simulink model "subsystem_118_bus"  (R2025b)
settings: Solver=ode45  StartTime=0.0  StopTime=Tstop  FixedStep=Ts  RelTol=1e-12  AbsTol=1e-12
values from neighbouring files (symbols this model uses):
  Imax = 15    [config_file.m]
  nominalInter =     [nominalInter.mat]
  nominalU =     [nominalU.mat]
  nominalY =     [nominalY.mat]
  sub = struct    [main_sub_118_bus.m]
  sys_j = sys_j(1:end-1)    [IBR_modelGenerator.m]
  sys_j_AA = sys_j    [modularMOR_main.m]
  sys_j_BT = sys_j    [modularMOR_main.m]
  Tstep_gfl = 0.1    [main_sub_118_bus.m]
  Tstep_gfm = 0.1    [main_sub_118_bus.m]
  w = 2*pi*50    (= 314.159265359)    [config_file.m]    (also in mirrorMimoWeightedFrequencyData.m = w(:); modularMOR_main.m = w(:).'; plotTest.m = w(:).')
undefined symbols (not defined in the file or in its folder): con_sub, linSys1, linSys2, linSys3
libraries: simulink x10
(part 2 of 6)

== system subsystem_118_bus/Linear 118 Bus ROM/Subsystem3/con13 ==
  In1 : Inport
  In2 : Inport  Port=2
  Constant : Constant  Value=con_subsystem.T
  Constant1 : Constant  Value=con_subsystem.T
  Mux : Mux  Inputs=2
  Selector : Selector  NumberOfDimensions=2  InputPortWidth=3  IndexOptions=Index vector (dialog),Select all  Indices=con_subsystem.reorder_v',1  OutputSizes=1,1
  Selector1 : Selector  InputPortWidth=con_subsystem.nbus  IndexOptions=Index vector (dialog)  Indices=con_subsystem.I_select{1}'  OutputSizes=1
  Selector2 : Selector  InputPortWidth=con_subsystem.nbus  IndexOptions=Index vector (dialog)  Indices=con_subsystem.I_select{3}'  OutputSizes=1
  T'x(v_bus_DQ) : Product  Multiplication=Matrix(*)
  Transpose : Math  Operator=transpose
  Tx(i_line_DQ) : Product  Multiplication=Matrix(*)
  branch RL dynamics : Subsystem
      mask Display: image('$imagefile'); % Use "Edit Image" on toolstrip to change.
  Out1 : Outport
  Out2 : Outport  Port=2
  wires:
  In2/1 -> Mux/2
  Selector2/1 -> Out2/1
  In1/1 -> Mux/1
  Selector1/1 -> Out1/1
  T'x(v_bus_DQ)/1 -> branch RL dynamics/1(v_diff_DQ)
  branch RL dynamics/1(i_line_DQ) -> Tx(i_line_DQ)/2
  Constant1/1 -> Tx(i_line_DQ)/1
  Transpose/1 -> T'x(v_bus_DQ)/1
  Constant/1 -> Transpose/1
  Tx(i_line_DQ)/1 -> Selector1/1, Selector2/1
  Selector/1 -> T'x(v_bus_DQ)/2
  Mux/1 -> Selector/1

== system subsystem_118_bus/Subsystem1/area1/branch RL dynamics ==
  v_diff_DQ : Inport
  " " : Integrator  InitialCondition=Subsystem.line.i_D  ContinuousStateAttributes='lineiD'
  -R/L : Gain  Gain=-Subsystem.line.r./Subsystem.line.l
  "-R/L " : Gain  Gain=-Subsystem.line.r./Subsystem.line.l
  1/L : Gain  Gain=1./Subsystem.line.l
  "1/L " : Gain  Gain=1./Subsystem.line.l
  Complex to Real-Imag : ComplexToRealImag
  Constant : Constant  Value=w
  Integrator1 : Integrator  InitialCondition=Subsystem.line.i_Q  ContinuousStateAttributes='lineiQ'
  Product : Product
  Product1 : Product
  Real-Imag to Complex : RealImagToComplex
  Sum2 : Sum  Inputs=+++
  Sum3 : Sum  Inputs=-++
  i_line_DQ : Outport
  wires:
  Sum2/1 -> " "/1
  Sum3/1 -> Integrator1/1
  Product/1 -> Sum2/3
  "1/L "/1 -> Sum3/2
  Product1/1 -> Sum3/1
  1/L/1 -> Sum2/2
  -R/L/1 -> Sum2/1
  "-R/L "/1 -> Sum3/3
  Integrator1/1 -> Real-Imag to Complex/2, Product/2, "-R/L "/1
  " "/1 -> Real-Imag to Complex/1, Product1/1, -R/L/1
  v_diff_DQ/1 -> Complex to Real-Imag/1
  Complex to Real-Imag/1 -> 1/L/1
  Complex to Real-Imag/2 -> "1/L "/1
  Real-Imag to Complex/1 -> i_line_DQ/1
  Constant/1 -> Product1/2, Product/1

== system subsystem_118_bus/Subsystem1/area1/bus reordering ==
  In1 : Inport
  In2 : Inport  Port=2
  Mux : Mux  Inputs=2
  Selector : Selector  NumberOfDimensions=2  InputPortWidth=3  IndexOptions=Index vector (dialog),Select all  Indices=Subsystem.reordering',1  OutputSizes=1,1
  v_bus_DQ : Outport
  wires:
  In2/1 -> Mux/2
  In1/1 -> Mux/1
  Mux/1 -> Selector/1
  Selector/1 -> v_bus_DQ/1

== system subsystem_118_bus/Subsystem1/area1/ibr ==
  I_bus_DQ : Inport
  Inport : Inport  Port=2
  Inport1 : Inport  Port=3
  Inport2 : Inport  Port=4
  Inport3 : Inport  Port=5
  Complex to Real-Imag : ComplexToRealImag
  Mux : Mux  Inputs=2
  Mux1 : Mux  Inputs=2
  Real-Imag to Complex : RealImagToComplex
  gfl : Subsystem
      mask Display: image('$imagefile'); % Use "Edit Image" on toolstrip to change.
  gfm : Subsystem  Commented=on
      mask Display: image('$imagefile'); % Use "Edit Image" on toolstrip to change.
  ibr device selector : Selector  InputPortWidth=Subsystem.total_devices.ibr  IndexOptions=Index vector (dialog)  Indices=Subsystem.device_selector.ibr  OutputSizes=1
  "ibr device selector " : Selector  InputPortWidth=Subsystem.total_devices.ibr  IndexOptions=Index vector (dialog)  Indices=Subsystem.device_selector.ibr  OutputSizes=1
  v_ibr_DQ : Outport
  Pm : Outport  Port=2
  Vm : Outport  Port=3
  Pm1 : Outport  Port=4
  Vm1 : Outport  Port=5
  wires:
  [v_gfl_pv_D] -> Mux/1
  [v_gfl_pv_Q] -> Mux1/1
  gfl/2(v_gfl_pv_Q) -> [v_gfl_pv_Q]
  gfm/1(v_gfm_pv_D) -> [v_gfm_D]
  gfm/2(v_gfm_pv_Q) -> [v_gfm_Q]
  Mux/1 -> ibr device selector/1
  Mux1/1 -> "ibr device selector "/1
  ibr device selector/1 -> Real-Imag to Complex/1
  "ibr device selector "/1 -> Real-Imag to Complex/2
  I_bus_DQ/1 -> Complex to Real-Imag/1
  Real-Imag to Complex/1 -> v_ibr_DQ/1
  Complex to Real-Imag/2 -> gfm/2(i_bus_Q), gfl/2(i_bus_Q)
  Complex to Real-Imag/1 -> gfm/1(i_bus_D), gfl/1(i_bus_D)
  gfl/1(vgfl_pv_D) -> [v_gfl_pv_D]
  [v_gfm_D] -> Mux/2
  [v_gfm_Q] -> Mux1/2
  Inport/1 -> gfl/3(Inport)
  Inport1/1 -> gfl/4(Inport1)
  gfl/4(Outport1) -> Vm/1
  gfl/3(Outport) -> Pm/1
  gfm/3(Outport) -> Pm1/1
  gfm/4(Outport1) -> Vm1/1
  Inport3/1 -> gfm/4(Inport1)
  Inport2/1 -> gfm/3(Inport)

== system subsystem_118_bus/Subsystem1/area1/non_ibr ==
  i_bus_DQ : Inport
  Complex to Real-Imag : ComplexToRealImag
  Mux : Mux  Inputs=3
  Mux1 : Mux  Inputs=3
  Real-Imag to Complex : RealImagToComplex
  floating buses : Subsystem
      mask Display: image('$imagefile'); % Use "Edit Image" on toolstrip to change.
  infinite bus : Subsystem  Commented=on
      mask Display: image('$imagefile'); % Use "Edit Image" on toolstrip to change.
  load buses : Subsystem
      mask Display: image('$imagefile'); % Use "Edit Image" on toolstrip to change.
  nonibr device selector : Selector  InputPortWidth=Subsystem.total_devices.nonibr  IndexOptions=Index vector (dialog)  Indices=Subsystem.device_selector.nonibr  OutputSizes=1
  "nonibr device selector " : Selector  InputPortWidth=Subsystem.total_devices.nonibr  IndexOptions=Index vector (dialog)  Indices=Subsystem.device_selector.nonibr  OutputSizes=1
  v_nonibr_DQ : Outport
  wires:
  infinite bus/1(Out1) -> [v_inf_D]
  infinite bus/2(Out2) -> [v_inf_Q]
  floating buses/1(v_float_D) -> [v_float_D]
  floating buses/2(v_float_Q) -> [v_float_Q]
  [v_inf_D] -> Mux/1
  Mux1/1 -> "nonibr device selector "/1
  [v_float_Q] -> Mux1/2
  [v_inf_Q] -> Mux1/1
  [v_float_D] -> Mux/2
  Mux/1 -> nonibr device selector/1
  nonibr device selector/1 -> Real-Imag to Complex/1
  "nonibr device selector "/1 -> Real-Imag to Complex/2
  Real-Imag to Complex/1 -> v_nonibr_DQ/1
  i_bus_DQ/1 -> Complex to Real-Imag/1
  Complex to Real-Imag/1 -> load buses/1(In1), floating buses/1(In1)
  Complex to Real-Imag/2 -> load buses/2(In2), floating buses/2(In2)
  load buses/2(Out2) -> [v_load_Q]
  load buses/1(Out1) -> [v_load_D]
  [v_load_D] -> Mux/3
  [v_load_Q] -> Mux1/3

== system subsystem_118_bus/Subsystem1/con12/branch RL dynamics ==
  v_diff_DQ : Inport
  " " : Integrator  InitialCondition=con_subsystem.line.i_D  ContinuousStateAttributes='lineiD'
  -R/L : Gain  Gain=-con_subsystem.line.r./con_subsystem.line.l
  "-R/L " : Gain  Gain=-con_subsystem.line.r./con_subsystem.line.l
  1/L : Gain  Gain=1./con_subsystem.line.l
  "1/L " : Gain  Gain=1./con_subsystem.line.l
  Complex to Real-Imag : ComplexToRealImag
  Constant : Constant  Value=w
  Integrator1 : Integrator  InitialCondition=con_subsystem.line.i_Q  ContinuousStateAttributes='lineiQ'
  Product : Product
  Product1 : Product
  Real-Imag to Complex : RealImagToComplex
  Sum2 : Sum  Inputs=+++
  Sum3 : Sum  Inputs=-++
  i_line_DQ : Outport
  wires:
  Sum2/1 -> " "/1
  Sum3/1 -> Integrator1/1
  Product/1 -> Sum2/3
  "1/L "/1 -> Sum3/2
  Product1/1 -> Sum3/1
  1/L/1 -> Sum2/2
  -R/L/1 -> Sum2/1
  "-R/L "/1 -> Sum3/3
  Integrator1/1 -> Real-Imag to Complex/2, Product/2, "-R/L "/1
  " "/1 -> Real-Imag to Complex/1, Product1/1, -R/L/1
  v_diff_DQ/1 -> Complex to Real-Imag/1
  Complex to Real-Imag/1 -> 1/L/1
  Complex to Real-Imag/2 -> "1/L "/1
  Real-Imag to Complex/1 -> i_line_DQ/1
  Constant/1 -> Product1/2, Product/1

== system subsystem_118_bus/Subsystem2/area2/branch RL dynamics ==
  v_diff_DQ : Inport
  " " : Integrator  InitialCondition=Subsystem.line.i_D  ContinuousStateAttributes='lineiD'
  -R/L : Gain  Gain=-Subsystem.line.r./Subsystem.line.l
  "-R/L " : Gain  Gain=-Subsystem.line.r./Subsystem.line.l
  1/L : Gain  Gain=1./Subsystem.line.l
  "1/L " : Gain  Gain=1./Subsystem.line.l
  Complex to Real-Imag : ComplexToRealImag
  Constant : Constant  Value=w
  Integrator1 : Integrator  InitialCondition=Subsystem.line.i_Q  ContinuousStateAttributes='lineiQ'
  Product : Product
  Product1 : Product
  Real-Imag to Complex : RealImagToComplex
  Sum2 : Sum  Inputs=+++
  Sum3 : Sum  Inputs=-++
  i_line_DQ : Outport
  wires:
  Constant/1 -> Product/1, Product1/2
  Real-Imag to Complex/1 -> i_line_DQ/1
  Complex to Real-Imag/2 -> "1/L "/1
  Complex to Real-Imag/1 -> 1/L/1
  v_diff_DQ/1 -> Complex to Real-Imag/1
  " "/1 -> -R/L/1, Product1/1, Real-Imag to Complex/1
  Integrator1/1 -> "-R/L "/1, Product/2, Real-Imag to Complex/2
  "-R/L "/1 -> Sum3/3
  -R/L/1 -> Sum2/1
  1/L/1 -> Sum2/2
  Product1/1 -> Sum3/1
  "1/L "/1 -> Sum3/2
  Product/1 -> Sum2/3
  Sum3/1 -> Integrator1/1
  Sum2/1 -> " "/1

== system subsystem_118_bus/Subsystem2/area2/bus reordering ==
  In1 : Inport
  In2 : Inport  Port=2
  Mux : Mux  Inputs=2
  Selector : Selector  NumberOfDimensions=2  InputPortWidth=3  IndexOptions=Index vector (dialog),Select all  Indices=Subsystem.reordering',1  OutputSizes=1,1
  v_bus_DQ : Outport
  wires:
  Selector/1 -> v_bus_DQ/1
  Mux/1 -> Selector/1
  In1/1 -> Mux/1
  In2/1 -> Mux/2

== system subsystem_118_bus/Subsystem2/area2/ibr ==
  I_bus_DQ : Inport
  Inport : Inport  Port=2
  Inport1 : Inport  Port=3
  Inport2 : Inport  Port=4
  Inport3 : Inport  Port=5
  Complex to Real-Imag : ComplexToRealImag
  Mux : Mux  Inputs=2
  Mux1 : Mux  Inputs=2
  Real-Imag to Complex : RealImagToComplex
  gfl : Subsystem
      mask Display: image('$imagefile'); % Use "Edit Image" on toolstrip to change.
  gfm : Subsystem
      mask Display: image('$imagefile'); % Use "Edit Image" on toolstrip to change.
  ibr device selector : Selector  InputPortWidth=Subsystem.total_devices.ibr  IndexOptions=Index vector (dialog)  Indices=Subsystem.device_selector.ibr  OutputSizes=1
  "ibr device selector " : Selector  InputPortWidth=Subsystem.total_devices.ibr  IndexOptions=Index vector (dialog)  Indices=Subsystem.device_selector.ibr  OutputSizes=1
  v_ibr_DQ : Outport
  Pm : Outport  Port=2
  Vm : Outport  Port=3
  Pm1 : Outport  Port=4
  Vm1 : Outport  Port=5
  wires:
  [v_gfl_pv_D] -> Mux/1
  [v_gfl_pv_Q] -> Mux1/1
  gfl/2(v_gfl_pv_Q) -> [v_gfl_pv_Q]
  gfm/1(v_gfm_pv_D) -> [v_gfm_D]
  gfm/2(v_gfm_pv_Q) -> [v_gfm_Q]
  Mux/1 -> ibr device selector/1
  Mux1/1 -> "ibr device selector "/1
  ibr device selector/1 -> Real-Imag to Complex/1
  "ibr device selector "/1 -> Real-Imag to Complex/2
  I_bus_DQ/1 -> Complex to Real-Imag/1
  Real-Imag to Complex/1 -> v_ibr_DQ/1
  Complex to Real-Imag/2 -> gfm/2(i_bus_Q), gfl/2(i_bus_Q)
  Complex to Real-Imag/1 -> gfm/1(i_bus_D), gfl/1(i_bus_D)
  gfl/1(vgfl_pv_D) -> [v_gfl_pv_D]
  [v_gfm_D] -> Mux/2
  [v_gfm_Q] -> Mux1/2
  Inport/1 -> gfl/3(Inport)
  Inport1/1 -> gfl/4(Inport1)
  gfl/4(Outport1) -> Vm/1
  gfl/3(Outport) -> Pm/1
  gfm/3(Outport) -> Pm1/1
  gfm/4(Outport1) -> Vm1/1
  Inport3/1 -> gfm/4(Inport1)
  Inport2/1 -> gfm/3(Inport)

== system subsystem_118_bus/Subsystem2/area2/non_ibr ==
  i_bus_DQ : Inport
  Complex to Real-Imag : ComplexToRealImag
  Mux : Mux  Inputs=3
  Mux1 : Mux  Inputs=3
  Real-Imag to Complex : RealImagToComplex
  floating buses : Subsystem
      mask Display: image('$imagefile'); % Use "Edit Image" on toolstrip to change.
  infinite bus : Subsystem  Commented=on
      mask Display: image('$imagefile'); % Use "Edit Image" on toolstrip to change.
  load buses : Subsystem
      mask Display: image('$imagefile'); % Use "Edit Image" on toolstrip to change.
  nonibr device selector : Selector  InputPortWidth=Subsystem.total_devices.nonibr  IndexOptions=Index vector (dialog)  Indices=Subsystem.device_selector.nonibr  OutputSizes=1
  "nonibr device selector " : Selector  InputPortWidth=Subsystem.total_devices.nonibr  IndexOptions=Index vector (dialog)  Indices=Subsystem.device_selector.nonibr  OutputSizes=1
  v_nonibr_DQ : Outport
  wires:
  [v_load_Q] -> Mux1/3
  [v_load_D] -> Mux/3
  load buses/1(Out1) -> [v_load_D]
  load buses/2(Out2) -> [v_load_Q]
  Complex to Real-Imag/2 -> floating buses/2(In2), load buses/2(In2)
  Complex to Real-Imag/1 -> floating buses/1(In1), load buses/1(In1)
  i_bus_DQ/1 -> Complex to Real-Imag/1
  Real-Imag to Complex/1 -> v_nonibr_DQ/1
  "nonibr device selector "/1 -> Real-Imag to Complex/2
  nonibr device selector/1 -> Real-Imag to Complex/1
  Mux/1 -> nonibr device selector/1
  [v_float_D] -> Mux/2
  [v_inf_Q] -> Mux1/1
  [v_float_Q] -> Mux1/2
  Mux1/1 -> "nonibr device selector "/1
  [v_inf_D] -> Mux/1
  floating buses/2(v_float_Q) -> [v_float_Q]
  floating buses/1(v_float_D) -> [v_float_D]
  infinite bus/2(Out2) -> [v_inf_Q]
  infinite bus/1(Out1) -> [v_inf_D]

== system subsystem_118_bus/Subsystem2/con23/branch RL dynamics ==
  v_diff_DQ : Inport
  " " : Integrator  InitialCondition=con_subsystem.line.i_D  ContinuousStateAttributes='lineiD'
  -R/L : Gain  Gain=-con_subsystem.line.r./con_subsystem.line.l
  "-R/L " : Gain  Gain=-con_subsystem.line.r./con_subsystem.line.l
  1/L : Gain  Gain=1./con_subsystem.line.l
  "1/L " : Gain  Gain=1./con_subsystem.line.l
  Complex to Real-Imag : ComplexToRealImag
  Constant : Constant  Value=w
  Integrator1 : Integrator  InitialCondition=con_subsystem.line.i_Q  ContinuousStateAttributes='lineiQ'
  Product : Product
  Product1 : Product
  Real-Imag to Complex : RealImagToComplex
  Sum2 : Sum  Inputs=+++
  Sum3 : Sum  Inputs=-++
  i_line_DQ : Outport
  wires:
  Sum2/1 -> " "/1
  Sum3/1 -> Integrator1/1
  Product/1 -> Sum2/3
  "1/L "/1 -> Sum3/2
  Product1/1 -> Sum3/1
  1/L/1 -> Sum2/2
  -R/L/1 -> Sum2/1
  "-R/L "/1 -> Sum3/3
  Integrator1/1 -> Real-Imag to Complex/2, Product/2, "-R/L "/1
  " "/1 -> Real-Imag to Complex/1, Product1/1, -R/L/1
  v_diff_DQ/1 -> Complex to Real-Imag/1
  Complex to Real-Imag/1 -> 1/L/1
  Complex to Real-Imag/2 -> "1/L "/1
  Real-Imag to Complex/1 -> i_line_DQ/1
  Constant/1 -> Product1/2, Product/1

== system subsystem_118_bus/Subsystem3/area3/branch RL dynamics ==
  v_diff_DQ : Inport
  " " : Integrator  InitialCondition=Subsystem.line.i_D  ContinuousStateAttributes='lineiD'
  -R/L : Gain  Gain=-Subsystem.line.r./Subsystem.line.l
  "-R/L " : Gain  Gain=-Subsystem.line.r./Subsystem.line.l
  1/L : Gain  Gain=1./Subsystem.line.l
  "1/L " : Gain  Gain=1./Subsystem.line.l
  Complex to Real-Imag : ComplexToRealImag
  Constant : Constant  Value=w
  Integrator1 : Integrator  InitialCondition=Subsystem.line.i_Q  ContinuousStateAttributes='lineiQ'
  Product : Product
  Product1 : Product
  Real-Imag to Complex : RealImagToComplex
  Sum2 : Sum  Inputs=+++
  Sum3 : Sum  Inputs=-++
  i_line_DQ : Outport
  wires:
  Sum2/1 -> " "/1
  Sum3/1 -> Integrator1/1
  Product/1 -> Sum2/3
  "1/L "/1 -> Sum3/2
  Product1/1 -> Sum3/1
  1/L/1 -> Sum2/2
  -R/L/1 -> Sum2/1
  "-R/L "/1 -> Sum3/3
  Integrator1/1 -> Real-Imag to Complex/2, Product/2, "-R/L "/1
  " "/1 -> Real-Imag to Complex/1, Product1/1, -R/L/1
  v_diff_DQ/1 -> Complex to Real-Imag/1
  Complex to Real-Imag/1 -> 1/L/1
  Complex to Real-Imag/2 -> "1/L "/1
  Real-Imag to Complex/1 -> i_line_DQ/1
  Constant/1 -> Product1/2, Product/1

== system subsystem_118_bus/Subsystem3/area3/bus reordering ==
  In1 : Inport
  In2 : Inport  Port=2
  Mux : Mux  Inputs=2
  Selector : Selector  NumberOfDimensions=2  InputPortWidth=3  IndexOptions=Index vector (dialog),Select all  Indices=Subsystem.reordering',1  OutputSizes=1,1
  v_bus_DQ : Outport
  wires:
  In2/1 -> Mux/2
  In1/1 -> Mux/1
  Mux/1 -> Selector/1
  Selector/1 -> v_bus_DQ/1

== system subsystem_118_bus/Subsystem3/area3/ibr ==
  I_bus_DQ : Inport
  Inport : Inport  Port=2
  Inport1 : Inport  Port=3
  Inport2 : Inport  Port=4
  Inport3 : Inport  Port=5
  Complex to Real-Imag : ComplexToRealImag
  Mux : Mux  Inputs=2
  Mux1 : Mux  Inputs=2
  Real-Imag to Complex : RealImagToComplex
  gfl : Subsystem
      mask Display: image('$imagefile'); % Use "Edit Image" on toolstrip to change.
  gfm : Subsystem  Commented=on
      mask Display: image('$imagefile'); % Use "Edit Image" on toolstrip to change.
  ibr device selector : Selector  InputPortWidth=Subsystem.total_devices.ibr  IndexOptions=Index vector (dialog)  Indices=Subsystem.device_selector.ibr  OutputSizes=1
  "ibr device selector " : Selector  InputPortWidth=Subsystem.total_devices.ibr  IndexOptions=Index vector (dialog)  Indices=Subsystem.device_selector.ibr  OutputSizes=1
  v_ibr_DQ : Outport
  Pm : Outport  Port=2
  Vm : Outport  Port=3
  Pm1 : Outport  Port=4
  Vm1 : Outport  Port=5
  wires:
  [v_gfl_pv_D] -> Mux/1
  [v_gfl_pv_Q] -> Mux1/1
  gfl/2(v_gfl_pv_Q) -> [v_gfl_pv_Q]
  gfm/1(v_gfm_pv_D) -> [v_gfm_D]
  gfm/2(v_gfm_pv_Q) -> [v_gfm_Q]
  Mux/1 -> ibr device selector/1
  Mux1/1 -> "ibr device selector "/1
  ibr device selector/1 -> Real-Imag to Complex/1
  "ibr device selector "/1 -> Real-Imag to Complex/2
  I_bus_DQ/1 -> Complex to Real-Imag/1
  Real-Imag to Complex/1 -> v_ibr_DQ/1
  Complex to Real-Imag/2 -> gfm/2(i_bus_Q), gfl/2(i_bus_Q)
  Complex to Real-Imag/1 -> gfm/1(i_bus_D), gfl/1(i_bus_D)
  gfl/1(vgfl_pv_D) -> [v_gfl_pv_D]
  [v_gfm_D] -> Mux/2
  [v_gfm_Q] -> Mux1/2
  Inport/1 -> gfl/3(Inport)
  Inport1/1 -> gfl/4(Inport1)
  gfl/4(Outport1) -> Vm/1
  gfl/3(Outport) -> Pm/1
  gfm/3(Outport) -> Pm1/1
  gfm/4(Outport1) -> Vm1/1
  Inport3/1 -> gfm/4(Inport1)
  Inport2/1 -> gfm/3(Inport)

== system subsystem_118_bus/Subsystem3/area3/non_ibr ==
  i_bus_DQ : Inport
  Complex to Real-Imag : ComplexToRealImag
  Mux : Mux  Inputs=3
  Mux1 : Mux  Inputs=3
  Real-Imag to Complex : RealImagToComplex
  floating buses : Subsystem  Commented=on
      mask Display: image('$imagefile'); % Use "Edit Image" on toolstrip to change.
  infinite bus : Subsystem  Commented=on
      mask Display: image('$imagefile'); % Use "Edit Image" on toolstrip to change.
  load buses : Subsystem
      mask Display: image('$imagefile'); % Use "Edit Image" on toolstrip to change.
  nonibr device selector : Selector  InputPortWidth=Subsystem.total_devices.nonibr  IndexOptions=Index vector (dialog)  Indices=Subsystem.device_selector.nonibr  OutputSizes=1
  "nonibr device selector " : Selector  InputPortWidth=Subsystem.total_devices.nonibr  IndexOptions=Index vector (dialog)  Indices=Subsystem.device_selector.nonibr  OutputSizes=1
  v_nonibr_DQ : Outport
  wires:
  infinite bus/1(Out1) -> [v_inf_D]
  infinite bus/2(Out2) -> [v_inf_Q]
  floating buses/1(v_float_D) -> [v_float_D]
  floating buses/2(v_float_Q) -> [v_float_Q]
  [v_inf_D] -> Mux/1
  Mux1/1 -> "nonibr device selector "/1
  [v_float_Q] -> Mux1/2
  [v_inf_Q] -> Mux1/1
  [v_float_D] -> Mux/2
  Mux/1 -> nonibr device selector/1
  nonibr device selector/1 -> Real-Imag to Complex/1
  "nonibr device selector "/1 -> Real-Imag to Complex/2
  Real-Imag to Complex/1 -> v_nonibr_DQ/1
  i_bus_DQ/1 -> Complex to Real-Imag/1
  Complex to Real-Imag/1 -> load buses/1(In1), floating buses/1(In1)
  Complex to Real-Imag/2 -> load buses/2(In2), floating buses/2(In2)
  load buses/2(Out2) -> [v_load_Q]
  load buses/1(Out1) -> [v_load_D]
  [v_load_D] -> Mux/3
  [v_load_Q] -> Mux1/3

== system subsystem_118_bus/Subsystem3/con13/branch RL dynamics ==
  v_diff_DQ : Inport
  " " : Integrator  InitialCondition=con_subsystem.line.i_D  ContinuousStateAttributes='lineiD'
  -R/L : Gain  Gain=-con_subsystem.line.r./con_subsystem.line.l
  "-R/L " : Gain  Gain=-con_subsystem.line.r./con_subsystem.line.l
  1/L : Gain  Gain=1./con_subsystem.line.l
  "1/L " : Gain  Gain=1./con_subsystem.line.l
  Complex to Real-Imag : ComplexToRealImag
  Constant : Constant  Value=w
  Integrator1 : Integrator  InitialCondition=con_subsystem.line.i_Q  ContinuousStateAttributes='lineiQ'
  Product : Product
  Product1 : Product
  Real-Imag to Complex : RealImagToComplex
  Sum2 : Sum  Inputs=+++
  Sum3 : Sum  Inputs=-++
  i_line_DQ : Outport
  wires:
  Constant/1 -> Product/1, Product1/2
  Real-Imag to Complex/1 -> i_line_DQ/1
  Complex to Real-Imag/2 -> "1/L "/1
  Complex to Real-Imag/1 -> 1/L/1
  v_diff_DQ/1 -> Complex to Real-Imag/1
  " "/1 -> -R/L/1, Product1/1, Real-Imag to Complex/1
  Integrator1/1 -> "-R/L "/1, Product/2, Real-Imag to Complex/2
  "-R/L "/1 -> Sum3/3
  -R/L/1 -> Sum2/1
  1/L/1 -> Sum2/2
  Product1/1 -> Sum3/1
  "1/L "/1 -> Sum3/2
  Product/1 -> Sum2/3
  Sum3/1 -> Integrator1/1
  Sum2/1 -> " "/1

== system subsystem_118_bus/Linear 118 Bus FOM/Subsystem3/area3/branch RL dynamics ==
  v_diff_DQ : Inport
  " " : Integrator  InitialCondition=Subsystem.line.i_D  ContinuousStateAttributes='lineiD'
  -R/L : Gain  Gain=-Subsystem.line.r./Subsystem.line.l
  "-R/L " : Gain  Gain=-Subsystem.line.r./Subsystem.line.l
  1/L : Gain  Gain=1./Subsystem.line.l
  "1/L " : Gain  Gain=1./Subsystem.line.l
  Complex to Real-Imag : ComplexToRealImag
  Constant : Constant  Value=w
  Integrator1 : Integrator  InitialCondition=Subsystem.line.i_Q  ContinuousStateAttributes='lineiQ'
  Product : Product
  Product1 : Product
  Real-Imag to Complex : RealImagToComplex
  Sum2 : Sum  Inputs=+++
  Sum3 : Sum  Inputs=-++
  i_line_DQ : Outport
  wires:
  Sum2/1 -> " "/1
  Sum3/1 -> Integrator1/1
  Product/1 -> Sum2/3
  "1/L "/1 -> Sum3/2
  Product1/1 -> Sum3/1
  1/L/1 -> Sum2/2
  -R/L/1 -> Sum2/1
  "-R/L "/1 -> Sum3/3
  Integrator1/1 -> Real-Imag to Complex/2, Product/2, "-R/L "/1
  " "/1 -> Real-Imag to Complex/1, Product1/1, -R/L/1
  v_diff_DQ/1 -> Complex to Real-Imag/1
  Complex to Real-Imag/1 -> 1/L/1
  Complex to Real-Imag/2 -> "1/L "/1
  Real-Imag to Complex/1 -> i_line_DQ/1
  Constant/1 -> Product1/2, Product/1

== system subsystem_118_bus/Linear 118 Bus FOM/Subsystem3/area3/bus reordering ==
  In1 : Inport
  In2 : Inport  Port=2
  Mux : Mux  Inputs=2
  Selector : Selector  NumberOfDimensions=2  InputPortWidth=3  IndexOptions=Index vector (dialog),Select all  Indices=Subsystem.reordering',1  OutputSizes=1,1
  v_bus_DQ : Outport
  wires:
  In2/1 -> Mux/2
  In1/1 -> Mux/1
  Mux/1 -> Selector/1
  Selector/1 -> v_bus_DQ/1

== system subsystem_118_bus/Linear 118 Bus FOM/Subsystem3/area3/ibr ==
  I_bus_DQ : Inport
  Inport : Inport  Port=2
  Inport1 : Inport  Port=3
  Inport2 : Inport  Port=4
  Inport3 : Inport  Port=5
  Complex to Real-Imag : ComplexToRealImag
  Mux : Mux  Inputs=2
  Mux1 : Mux  Inputs=2
  Real-Imag to Complex : RealImagToComplex
  gfl : Subsystem
      mask Display: image('$imagefile'); % Use "Edit Image" on toolstrip to change.
  gfm : Subsystem  Commented=on
      mask Display: image('$imagefile'); % Use "Edit Image" on toolstrip to change.
  ibr device selector : Selector  InputPortWidth=Subsystem.total_devices.ibr  IndexOptions=Index vector (dialog)  Indices=Subsystem.device_selector.ibr  OutputSizes=1
  "ibr device selector " : Selector  InputPortWidth=Subsystem.total_devices.ibr  IndexOptions=Index vector (dialog)  Indices=Subsystem.device_selector.ibr  OutputSizes=1
  v_ibr_DQ : Outport
  Pm : Outport  Port=2
  Vm : Outport  Port=3
  Pm1 : Outport  Port=4
  Vm1 : Outport  Port=5
  wires:
  [v_gfl_pv_D] -> Mux/1
  [v_gfl_pv_Q] -> Mux1/1
  gfl/2(v_gfl_pv_Q) -> [v_gfl_pv_Q]
  gfm/1(v_gfm_pv_D) -> [v_gfm_D]
  gfm/2(v_gfm_pv_Q) -> [v_gfm_Q]
  Mux/1 -> ibr device selector/1
  Mux1/1 -> "ibr device selector "/1
  ibr device selector/1 -> Real-Imag to Complex/1
  "ibr device selector "/1 -> Real-Imag to Complex/2
  I_bus_DQ/1 -> Complex to Real-Imag/1
  Real-Imag to Complex/1 -> v_ibr_DQ/1
  Complex to Real-Imag/2 -> gfm/2(i_bus_Q), gfl/2(i_bus_Q)
  Complex to Real-Imag/1 -> gfm/1(i_bus_D), gfl/1(i_bus_D)
  gfl/1(vgfl_pv_D) -> [v_gfl_pv_D]
  [v_gfm_D] -> Mux/2
  [v_gfm_Q] -> Mux1/2
  Inport/1 -> gfl/3(Inport)
  Inport1/1 -> gfl/4(Inport1)
  gfl/4(Outport1) -> Vm/1
  gfl/3(Outport) -> Pm/1
  gfm/3(Outport) -> Pm1/1
  gfm/4(Outport1) -> Vm1/1
  Inport3/1 -> gfm/4(Inport1)
  Inport2/1 -> gfm/3(Inport)

== system subsystem_118_bus/Linear 118 Bus FOM/Subsystem3/area3/non_ibr ==
  i_bus_DQ : Inport
  Complex to Real-Imag : ComplexToRealImag
  Mux : Mux  Inputs=3
  Mux1 : Mux  Inputs=3
  Real-Imag to Complex : RealImagToComplex
  floating buses : Subsystem  Commented=on
      mask Display: image('$imagefile'); % Use "Edit Image" on toolstrip to change.
  infinite bus : Subsystem  Commented=on
      mask Display: image('$imagefile'); % Use "Edit Image" on toolstrip to change.
  load buses : Subsystem
      mask Display: image('$imagefile'); % Use "Edit Image" on toolstrip to change.
  nonibr device selector : Selector  InputPortWidth=Subsystem.total_devices.nonibr  IndexOptions=Index vector (dialog)  Indices=Subsystem.device_selector.nonibr  OutputSizes=1
  "nonibr device selector " : Selector  InputPortWidth=Subsystem.total_devices.nonibr  IndexOptions=Index vector (dialog)  Indices=Subsystem.device_selector.nonibr  OutputSizes=1
  v_nonibr_DQ : Outport
  wires:
  infinite bus/1(Out1) -> [v_inf_D]
  infinite bus/2(Out2) -> [v_inf_Q]
  floating buses/1(v_float_D) -> [v_float_D]
  floating buses/2(v_float_Q) -> [v_float_Q]
  [v_inf_D] -> Mux/1
  Mux1/1 -> "nonibr device selector "/1
  [v_float_Q] -> Mux1/2
  [v_inf_Q] -> Mux1/1
  [v_float_D] -> Mux/2
  Mux/1 -> nonibr device selector/1
  nonibr device selector/1 -> Real-Imag to Complex/1
  "nonibr device selector "/1 -> Real-Imag to Complex/2
  Real-Imag to Complex/1 -> v_nonibr_DQ/1
  i_bus_DQ/1 -> Complex to Real-Imag/1
  Complex to Real-Imag/1 -> load buses/1(In1), floating buses/1(In1)
  Complex to Real-Imag/2 -> load buses/2(In2), floating buses/2(In2)
  load buses/2(Out2) -> [v_load_Q]
  load buses/1(Out1) -> [v_load_D]
  [v_load_D] -> Mux/3
  [v_load_Q] -> Mux1/3

== system subsystem_118_bus/Linear 118 Bus FOM/Subsystem3/con13/branch RL dynamics ==
  v_diff_DQ : Inport
  " " : Integrator  InitialCondition=con_subsystem.line.i_D  ContinuousStateAttributes='lineiD'
  -R/L : Gain  Gain=-con_subsystem.line.r./con_subsystem.line.l
  "-R/L " : Gain  Gain=-con_subsystem.line.r./con_subsystem.line.l
  1/L : Gain  Gain=1./con_subsystem.line.l
  "1/L " : Gain  Gain=1./con_subsystem.line.l
  Complex to Real-Imag : ComplexToRealImag
  Constant : Constant  Value=w
  Integrator1 : Integrator  InitialCondition=con_subsystem.line.i_Q  ContinuousStateAttributes='lineiQ'
  Product : Product
  Product1 : Product
  Real-Imag to Complex : RealImagToComplex
  Sum2 : Sum  Inputs=+++
  Sum3 : Sum  Inputs=-++
  i_line_DQ : Outport
  wires:
  Constant/1 -> Product/1, Product1/2
  Real-Imag to Complex/1 -> i_line_DQ/1
  Complex to Real-Imag/2 -> "1/L "/1
  Complex to Real-Imag/1 -> 1/L/1
  v_diff_DQ/1 -> Complex to Real-Imag/1
  " "/1 -> -R/L/1, Product1/1, Real-Imag to Complex/1
  Integrator1/1 -> "-R/L "/1, Product/2, Real-Imag to Complex/2
  "-R/L "/1 -> Sum3/3
  -R/L/1 -> Sum2/1
  1/L/1 -> Sum2/2
  Product1/1 -> Sum3/1
  "1/L "/1 -> Sum3/2
  Product/1 -> Sum2/3
  Sum3/1 -> Integrator1/1
  Sum2/1 -> " "/1

== system subsystem_118_bus/Linear 118 Bus ROM/Subsystem3/area3/branch RL dynamics ==
  v_diff_DQ : Inport
  " " : Integrator  InitialCondition=Subsystem.line.i_D  ContinuousStateAttributes='lineiD'
  -R/L : Gain  Gain=-Subsystem.line.r./Subsystem.line.l
  "-R/L " : Gain  Gain=-Subsystem.line.r./Subsystem.line.l
  1/L : Gain  Gain=1./Subsystem.line.l
  "1/L " : Gain  Gain=1./Subsystem.line.l
  Complex to Real-Imag : ComplexToRealImag
  Constant : Constant  Value=w
  Integrator1 : Integrator  InitialCondition=Subsystem.line.i_Q  ContinuousStateAttributes='lineiQ'
  Product : Product
  Product1 : Product
  Real-Imag to Complex : RealImagToComplex
  Sum2 : Sum  Inputs=+++
  Sum3 : Sum  Inputs=-++
  i_line_DQ : Outport
  wires:
  Sum2/1 -> " "/1
  Sum3/1 -> Integrator1/1
  Product/1 -> Sum2/3
  "1/L "/1 -> Sum3/2
  Product1/1 -> Sum3/1
  1/L/1 -> Sum2/2
  -R/L/1 -> Sum2/1
  "-R/L "/1 -> Sum3/3
  Integrator1/1 -> Real-Imag to Complex/2, Product/2, "-R/L "/1
  " "/1 -> Real-Imag to Complex/1, Product1/1, -R/L/1
  v_diff_DQ/1 -> Complex to Real-Imag/1
  Complex to Real-Imag/1 -> 1/L/1
  Complex to Real-Imag/2 -> "1/L "/1
  Real-Imag to Complex/1 -> i_line_DQ/1
  Constant/1 -> Product1/2, Product/1

== system subsystem_118_bus/Linear 118 Bus ROM/Subsystem3/area3/bus reordering ==
  In1 : Inport
  In2 : Inport  Port=2
  Mux : Mux  Inputs=2
  Selector : Selector  NumberOfDimensions=2  InputPortWidth=3  IndexOptions=Index vector (dialog),Select all  Indices=Subsystem.reordering',1  OutputSizes=1,1
  v_bus_DQ : Outport
  wires:
  In2/1 -> Mux/2
  In1/1 -> Mux/1
  Mux/1 -> Selector/1
  Selector/1 -> v_bus_DQ/1

== system subsystem_118_bus/Linear 118 Bus ROM/Subsystem3/area3/ibr ==
  I_bus_DQ : Inport
  Inport : Inport  Port=2
  Inport1 : Inport  Port=3
  Inport2 : Inport  Port=4
  Inport3 : Inport  Port=5
  Complex to Real-Imag : ComplexToRealImag
  Mux : Mux  Inputs=2
  Mux1 : Mux  Inputs=2
  Real-Imag to Complex : RealImagToComplex
  gfl : Subsystem
      mask Display: image('$imagefile'); % Use "Edit Image" on toolstrip to change.
  gfm : Subsystem  Commented=on
      mask Display: image('$imagefile'); % Use "Edit Image" on toolstrip to change.
  ibr device selector : Selector  InputPortWidth=Subsystem.total_devices.ibr  IndexOptions=Index vector (dialog)  Indices=Subsystem.device_selector.ibr  OutputSizes=1
  "ibr device selector " : Selector  InputPortWidth=Subsystem.total_devices.ibr  IndexOptions=Index vector (dialog)  Indices=Subsystem.device_selector.ibr  OutputSizes=1
  v_ibr_DQ : Outport
  Pm : Outport  Port=2
  Vm : Outport  Port=3
  Pm1 : Outport  Port=4
  Vm1 : Outport  Port=5
  wires:
  [v_gfl_pv_D] -> Mux/1
  [v_gfl_pv_Q] -> Mux1/1
  gfl/2(v_gfl_pv_Q) -> [v_gfl_pv_Q]
  gfm/1(v_gfm_pv_D) -> [v_gfm_D]
  gfm/2(v_gfm_pv_Q) -> [v_gfm_Q]
  Mux/1 -> ibr device selector/1
  Mux1/1 -> "ibr device selector "/1
  ibr device selector/1 -> Real-Imag to Complex/1
  "ibr device selector "/1 -> Real-Imag to Complex/2
  I_bus_DQ/1 -> Complex to Real-Imag/1
  Real-Imag to Complex/1 -> v_ibr_DQ/1
  Complex to Real-Imag/2 -> gfm/2(i_bus_Q), gfl/2(i_bus_Q)
  Complex to Real-Imag/1 -> gfm/1(i_bus_D), gfl/1(i_bus_D)
  gfl/1(vgfl_pv_D) -> [v_gfl_pv_D]
  [v_gfm_D] -> Mux/2
  [v_gfm_Q] -> Mux1/2
  Inport/1 -> gfl/3(Inport)
  Inport1/1 -> gfl/4(Inport1)
  gfl/4(Outport1) -> Vm/1
  gfl/3(Outport) -> Pm/1
  gfm/3(Outport) -> Pm1/1
  gfm/4(Outport1) -> Vm1/1
  Inport3/1 -> gfm/4(Inport1)
  Inport2/1 -> gfm/3(Inport)

== system subsystem_118_bus/Linear 118 Bus ROM/Subsystem3/area3/non_ibr ==
  i_bus_DQ : Inport
  Complex to Real-Imag : ComplexToRealImag
  Mux : Mux  Inputs=3
  Mux1 : Mux  Inputs=3
  Real-Imag to Complex : RealImagToComplex
  floating buses : Subsystem  Commented=on
      mask Display: image('$imagefile'); % Use "Edit Image" on toolstrip to change.
  infinite bus : Subsystem  Commented=on
      mask Display: image('$imagefile'); % Use "Edit Image" on toolstrip to change.
  load buses : Subsystem
      mask Display: image('$imagefile'); % Use "Edit Image" on toolstrip to change.
  nonibr device selector : Selector  InputPortWidth=Subsystem.total_devices.nonibr  IndexOptions=Index vector (dialog)  Indices=Subsystem.device_selector.nonibr  OutputSizes=1
  "nonibr device selector " : Selector  InputPortWidth=Subsystem.total_devices.nonibr  IndexOptions=Index vector (dialog)  Indices=Subsystem.device_selector.nonibr  OutputSizes=1
  v_nonibr_DQ : Outport
  wires:
  infinite bus/1(Out1) -> [v_inf_D]
  infinite bus/2(Out2) -> [v_inf_Q]
  floating buses/1(v_float_D) -> [v_float_D]
  floating buses/2(v_float_Q) -> [v_float_Q]
  [v_inf_D] -> Mux/1
  Mux1/1 -> "nonibr device selector "/1
  [v_float_Q] -> Mux1/2
  [v_inf_Q] -> Mux1/1
  [v_float_D] -> Mux/2
  Mux/1 -> nonibr device selector/1
  nonibr device selector/1 -> Real-Imag to Complex/1
  "nonibr device selector "/1 -> Real-Imag to Complex/2
  Real-Imag to Complex/1 -> v_nonibr_DQ/1
  i_bus_DQ/1 -> Complex to Real-Imag/1
  Complex to Real-Imag/1 -> load buses/1(In1), floating buses/1(In1)
  Complex to Real-Imag/2 -> load buses/2(In2), floating buses/2(In2)
  load buses/2(Out2) -> [v_load_Q]
  load buses/1(Out1) -> [v_load_D]
  [v_load_D] -> Mux/3
  [v_load_Q] -> Mux1/3

== system subsystem_118_bus/Linear 118 Bus ROM/Subsystem3/con13/branch RL dynamics ==
  v_diff_DQ : Inport
  " " : Integrator  InitialCondition=con_subsystem.line.i_D  ContinuousStateAttributes='lineiD'
  -R/L : Gain  Gain=-con_subsystem.line.r./con_subsystem.line.l
  "-R/L " : Gain  Gain=-con_subsystem.line.r./con_subsystem.line.l
  1/L : Gain  Gain=1./con_subsystem.line.l
  "1/L " : Gain  Gain=1./con_subsystem.line.l
  Complex to Real-Imag : ComplexToRealImag
  Constant : Constant  Value=w
  Integrator1 : Integrator  InitialCondition=con_subsystem.line.i_Q  ContinuousStateAttributes='lineiQ'
  Product : Product
  Product1 : Product
  Real-Imag to Complex : RealImagToComplex
  Sum2 : Sum  Inputs=+++
  Sum3 : Sum  Inputs=-++
  i_line_DQ : Outport
  wires:
  Constant/1 -> Product/1, Product1/2
  Real-Imag to Complex/1 -> i_line_DQ/1
  Complex to Real-Imag/2 -> "1/L "/1
  Complex to Real-Imag/1 -> 1/L/1
  v_diff_DQ/1 -> Complex to Real-Imag/1
  " "/1 -> -R/L/1, Product1/1, Real-Imag to Complex/1
  Integrator1/1 -> "-R/L "/1, Product/2, Real-Imag to Complex/2
  "-R/L "/1 -> Sum3/3
  -R/L/1 -> Sum2/1
  1/L/1 -> Sum2/2
  Product1/1 -> Sum3/1
  "1/L "/1 -> Sum3/2
  Product/1 -> Sum2/3
  Sum3/1 -> Integrator1/1
  Sum2/1 -> " "/1

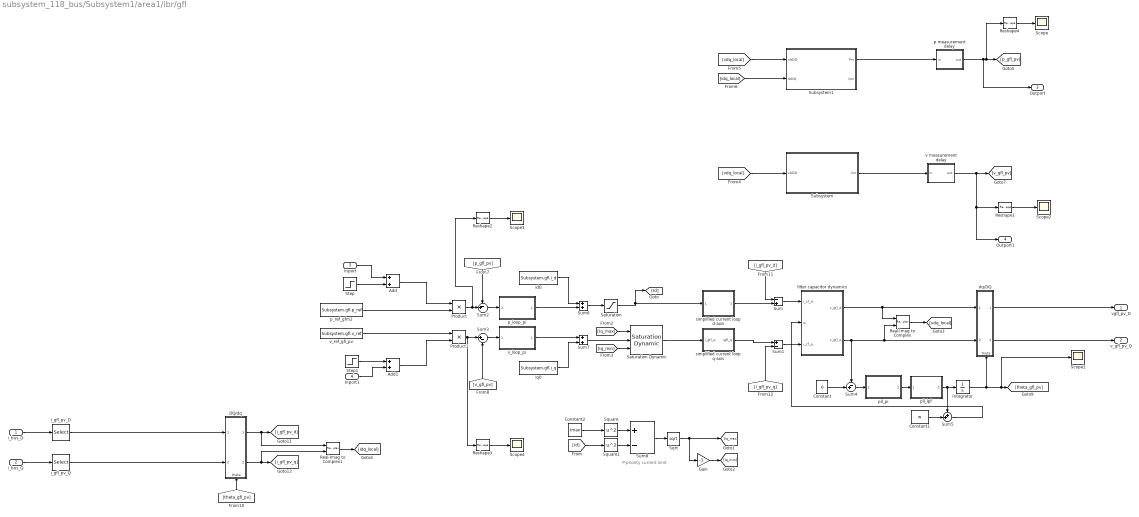
== system subsystem_118_bus/Subsystem1/area1/ibr/gfl ==
  note: P-priority current limit
  i_bus_D : Inport
  i_bus_Q : Inport  Port=2
  Inport : Inport  Port=3
  Inport1 : Inport  Port=4
  Add : Sum
  Add1 : Sum
  Constant : Constant  Value=0
  Constant1 : Constant  Value=w
  Constant2 : Constant  Value=Imax
  DQ/dq : Subsystem
      settings: PortSchema="{\"entries\":[{\"content\":{\"sides\":[{\"content\":{\"connectorIds\":[\"In1\",\"In2\"]},\"type\":\"ConnectorPlacement.EquallySpacedRectSide\",\"uuid\":\"6aba5a73-e9d3-440a-9da8-5b4060b79a22\"},{\"content\":{\"connectorIds\":[\"Out1\",\"Out2\"],\"side\":\"RIGHT\"},\"type\":\"ConnectorPlacement.EquallySpacedRectSide\",\"uuid\":\"fb100e33-0f2b-446b-b234-6a01cff1cf94\"},{\"content\":{\"connectorIds\":[],\"side\":\"TOP\"},\"type\":\"ConnectorPlacement.EquallySpacedRectSide\",\"uuid\":\"cb346bab-8363-4920-b8bd-1af08716b150\"},{\"content\":{\"connectorIds\":[\"In3\"],\"side\":\"BOTTOM\"},\"type\":\"ConnectorPlacement.EquallySpacedRectSide\",\"uuid\":\"daf67601-a33f-44c6-bbbf-d32eadf086e5\"},{\"content\":{\"connectorIds\":[],\"side\":\"HIDDEN\"},\"type\":\"ConnectorPlacement.EquallySpacedRectSide\",\"uuid\":\"157b31a2-d1ec-4854-8b21-1495795af5ef\"}]},\"type\":\"ConnectorPlacement.EquallySpacedConnector\",\"uuid\":\"bdcd0df2-60ef-4202-9e13-560935cf5e64\"}],\"packageUris\":[\"http://schema.mathworks.com/mf0/Connector/R2020b\"],\"version\":\"1.0\"}"
      mask Display: image('$imagefile'); % Use "Edit Image" on toolstrip to change.
  Gain : Gain  Gain=-1
  Integrator : Integrator  InitialCondition=Subsystem.gfl.theta  ContinuousStateAttributes='gfl_osc'
  Product : Product
  Product1 : Product
  Real-Imag to Complex : RealImagToComplex
  Real-Imag to Complex1 : RealImagToComplex
  Reshape{1..4} (4 alike) : Reshape
  Saturation : Saturate  UpperLimit=Imax  LowerLimit=-Imax
  Saturation Dynamic : simulink/Discontinuities/Saturation Dynamic  OutMin=[]  OutMax=[]  OutDataTypeStr=Inherit: Same as second input  OutDataType=fixdt(1, 16)  OutScaling=2^-10  DoSatur=off
  Scope{,1..4} (5 alike) : Scope
      Scope settings: ActiveDisplayYMinimum=-1  ActiveDisplayYMaximum=1  DataLoggingVariableName=pm_gfl  DataLoggingSaveFormat=Structure
      Scope1 settings: DataLoggingVariableName=thetagflwnd  DataLoggingSaveFormat=Structure
      Scope2 settings: ActiveDisplayYMinimum=-1  ActiveDisplayYMaximum=1  DataLoggingVariableName=vm_gfl  DataLoggingSaveFormat=Structure
      Scope3 settings: ActiveDisplayYMinimum=0.75  ActiveDisplayYMaximum=0.95  DataLoggingVariableName=pr_gfl  DataLoggingSaveFormat=Structure
      Scope4 settings: ActiveDisplayYMinimum=1.02188  ActiveDisplayYMaximum=1.05312  DataLoggingVariableName=vr_gfl  DataLoggingSaveFormat=Structure
  Sqrt : Sqrt
  Square : Math  Operator=square
  Square1 : Math  Operator=square
  Step : Step  Time=Tstep_gfl  Before=Subsystem.P_before_gfl  After=Subsystem.P_after_gfl  SampleTime=0
  Step1 : Step  Time=Tstep_gfl  Before=Subsystem.V_before_gfl  After=Subsystem.V_after_gfl  SampleTime=0
  Subsystem : Subsystem
      mask Display: image('$imagefile'); % Use "Edit Image" on toolstrip to change.
  Subsystem1 : Subsystem
      mask Display: image('$imagefile'); % Use "Edit Image" on toolstrip to change.
  Sum : Sum  Inputs=-+
  Sum1 : Sum  Inputs=+-
  Sum2 : Sum  Inputs=-+|
  Sum3 : Sum  Inputs=|+-
  Sum4 : Sum  Inputs=-+|
  Sum5 : Sum  Inputs=++|
  Sum6 : Sum
  Sum7 : Sum
  Sum8 : Sum  Inputs=+-
  dq/DQ : Subsystem
      settings: PortSchema="{\"entries\":[{\"content\":{\"sides\":[{\"content\":{\"connectorIds\":[\"In1\",\"In2\"]},\"type\":\"ConnectorPlacement.EquallySpacedRectSide\",\"uuid\":\"6aba5a73-e9d3-440a-9da8-5b4060b79a22\"},{\"content\":{\"connectorIds\":[\"Out1\",\"Out2\"],\"side\":\"RIGHT\"},\"type\":\"ConnectorPlacement.EquallySpacedRectSide\",\"uuid\":\"fb100e33-0f2b-446b-b234-6a01cff1cf94\"},{\"content\":{\"connectorIds\":[],\"side\":\"TOP\"},\"type\":\"ConnectorPlacement.EquallySpacedRectSide\",\"uuid\":\"cb346bab-8363-4920-b8bd-1af08716b150\"},{\"content\":{\"connectorIds\":[\"In3\"],\"side\":\"BOTTOM\"},\"type\":\"ConnectorPlacement.EquallySpacedRectSide\",\"uuid\":\"daf67601-a33f-44c6-bbbf-d32eadf086e5\"},{\"content\":{\"connectorIds\":[],\"side\":\"HIDDEN\"},\"type\":\"ConnectorPlacement.EquallySpacedRectSide\",\"uuid\":\"157b31a2-d1ec-4854-8b21-1495795af5ef\"}]},\"type\":\"ConnectorPlacement.EquallySpacedConnector\",\"uuid\":\"bdcd0df2-60ef-4202-9e13-560935cf5e64\"}],\"packageUris\":[\"http://schema.mathworks.com/mf0/Connector/R2020b\"],\"version\":\"1.0\"}"
      mask Display: image('$imagefile'); % Use "Edit Image" on toolstrip to change.
  filter capacitor dynamics : Subsystem
      mask Display: image('$imagefile'); % Use "Edit Image" on toolstrip to change.
  i_gfl_pv_D : Selector  InputPortWidth=size(Subsystem.sys_data,1)  IndexOptions=Index vector (dialog)  Indices=Subsystem.busnum.gfl  OutputSizes=1
  i_gfl_pv_Q : Selector  InputPortWidth=size(Subsystem.sys_data,1)  IndexOptions=Index vector (dialog)  Indices=Subsystem.busnum.gfl  OutputSizes=1
  id0 : Constant  Value=Subsystem.gfl.i_d
  iq0 : Constant  Value=Subsystem.gfl.i_q
  p measurement delay : Subsystem
      mask Display: image('$imagefile'); % Use "Edit Image" on toolstrip to change.
  p_loop_pi : Subsystem
      mask Display: image('$imagefile'); % Use "Edit Image" on toolstrip to change.
  p_ref_gfm2 : Constant  Value=Subsystem.gfl.p_ref
  pll_lpf : Subsystem
      mask Display: image('$imagefile'); % Use "Edit Image" on toolstrip to change.
  pll_pi : Subsystem
      mask Display: image('$imagefile'); % Use "Edit Image" on toolstrip to change.
  simplified current loop d-axis : Subsystem
      mask Display: image('$imagefile'); % Use "Edit Image" on toolstrip to change.
  simplified current loop q-axis : Subsystem
      mask Display: image('$imagefile'); % Use "Edit Image" on toolstrip to change.
  v measurement delay : Subsystem
      mask Display: image('$imagefile'); % Use "Edit Image" on toolstrip to change.
  v_loop_pi : Subsystem
      mask Display: image('$imagefile'); % Use "Edit Image" on toolstrip to change.
  v_ref_gfl_pv : Constant  Value=Subsystem.gfl.v_ref
  vgfl_pv_D : Outport
  v_gfl_pv_Q : Outport  Port=2
  Outport : Outport  Port=3
  Outport1 : Outport  Port=4
  wires:
  pll_lpf/1(LPF_output) -> Sum5/1, Integrator/1
  Constant/1 -> Sum4/2
  filter capacitor dynamics/1(v_gfl_d) -> dq/DQ/1(d-quantity), Real-Imag to Complex/1
  v measurement delay/1(out) -> Reshape1/1, Outport1/1, [v_gfl_pv]
  filter capacitor dynamics/2(v_gfl_q) -> Real-Imag to Complex/2, dq/DQ/2(q-quantity), Sum4/1
  [p_gfl_pv] -> Sum2/1
  Sum1/1 -> filter capacitor dynamics/3(i_cf_q)
  Sum4/1 -> pll_pi/1("  ")
  Sum5/1 -> filter capacitor dynamics/2(w)
  dq/DQ/1(D-quantity) -> vgfl_pv_D/1
  Sum2/1 -> p_loop_pi/1("  ")
  p measurement delay/1(out) -> Outport/1, Reshape4/1, [p_gfl_pv]
  Constant1/1 -> Sum5/2
  Sum3/1 -> v_loop_pi/1("  ")
  [i_gfl_pv_d] -> Sum/1
  Sum/1 -> filter capacitor dynamics/1(i_cf_d)
  [i_gfl_pv_q] -> Sum1/2
  [theta_gfl_pv] -> DQ/dq/3(theta)
  pll_pi/1(" ") -> pll_lpf/1(LPF_input)
  [v_gfl_pv] -> Sum3/2
  i_bus_Q/1 -> i_gfl_pv_Q/1
  i_bus_D/1 -> i_gfl_pv_D/1
  p_loop_pi/1(" ") -> Sum6/2
  v_loop_pi/1(" ") -> Sum7/1
  iq0/1 -> Sum7/2
  id0/1 -> Sum6/1
  Sum6/1 -> Saturation/1
  Integrator/1 -> Scope1/1, [theta_gfl_pv], dq/DQ/3(theta)
  Reshape4/1 -> Scope/1
  Reshape1/1 -> Scope2/1
  [Id] -> Square1/1
  Gain/1 -> [Iq_min]
  Constant2/1 -> Square/1
  Square/1 -> Sum8/1
  Sqrt/1 -> [Iq_max], Gain/1
  Square1/1 -> Sum8/2
  Sum8/1 -> Sqrt/1
  Saturation/1 -> simplified current loop d-axis/1(" "), [Id]
  Sum7/1 -> Saturation Dynamic/2
  [Iq_max] -> Saturation Dynamic/1
  [Iq_min] -> Saturation Dynamic/3
  simplified current loop d-axis/1("  ") -> Sum/2
  Saturation Dynamic/1 -> simplified current loop q-axis/1(i_gfl_q)
  simplified current loop q-axis/1(igfl_q) -> Sum1/1
  [vdq_local] -> Subsystem/1(vbDQ)
  [vdq_local] -> Subsystem1/1(vbDQ)
  [idq_local] -> Subsystem1/2(IbDQ)
  Real-Imag to Complex/1 -> [vdq_local]
  DQ/dq/1(d_quantity) -> Real-Imag to Complex1/1, [i_gfl_pv_d]
  DQ/dq/2(q_quantity) -> Real-Imag to Complex1/2, [i_gfl_pv_q]
  Real-Imag to Complex1/1 -> [idq_local]
  dq/DQ/2(Q-quantity) -> v_gfl_pv_Q/1
  Subsystem/1(Vm) -> v measurement delay/1(in)
  Subsystem1/1(Pm) -> p measurement delay/1(in)
  p_ref_gfm2/1 -> Product/2
  v_ref_gfl_pv/1 -> Product1/1
  Reshape2/1 -> Scope3/1
  Product/1 -> Reshape2/1, Sum2/2
  Reshape3/1 -> Scope4/1
  Product1/1 -> Sum3/1, Reshape3/1
  Step/1 -> Add/2
  Add/1 -> Product/1
  Step1/1 -> Add1/1
  Add1/1 -> Product1/2
  Inport/1 -> Add/1
  Inport1/1 -> Add1/2
  i_gfl_pv_D/1 -> DQ/dq/1(D_quantity)
  i_gfl_pv_Q/1 -> DQ/dq/2(Q_quantity)
